simulink model "PoleCart"  (R2025a)
settings: Solver=ode23s  StartTime=0.0  StopTime=Tf  RelTol=1e-3  AbsTol=1e-3  EnableMultiTasking=on
model workspace (MAT data in the model file):
  Max_Trq = 10
values from neighbouring files (symbols this model uses):
  AncleDegLowerLim = -45    [PoleCart_ini.m]    (also in initialize_Parameters.m = Simulink.Parameter)
  AncleDegUpperLim = 45    [PoleCart_ini.m]    (also in initialize_Parameters.m = Simulink.Parameter)
  BallUnderFootRad = 1e-2    (= 0.01)    [PoleCart_ini.m]    (also in initialize_Parameters.m = Simulink.Parameter)
  FootX = 0.1    [PoleCart_ini.m]    (also in initialize_Parameters.m = Simulink.Parameter)
  FootY = 0.25    [PoleCart_ini.m]    (also in initialize_Parameters.m = Simulink.Parameter)
  FootZ = 0.06    [PoleCart_ini.m]    (also in initialize_Parameters.m = Simulink.Parameter)
  InitialCondition = []    [initialize_Parameters.m]
  TibiaZ = 0.4    [PoleCart_ini.m]    (also in initialize_Parameters.m = Simulink.Parameter)
undefined symbols (not defined in the file or in its folder): X, Y, Z
libraries: sm_lib x24, nesl_utility x14, simulink x2, rllib x1
settings Model: Creator=naoki  LastModifiedBy=naoki
settings SolverCC: AutoScaleAbsTol=off  AlgebraicLoopSolver=TrustRegion  MaxZcPerStep=1.0
settings DataIOCC: LimitDataPoints=on  MaxDataPoints=10000
settings OptimizationCC: ReuseModelBlockBuffer=off  LifeSpan=inf
settings DebuggingCC: UnconnectedInputMsg=warning  UnconnectedOutputMsg=warning  UnconnectedLineMsg=warning  AllowSymbolicDim=off  SubsystemReferenceDiagnosticForUnitTest=warning  SFUnexpectedBacktrackingDiag=warning  SFNoUnconditionalDefaultTransitionDiag=warning  SFExecutionAtInitializationDiag=none  ArithmeticOperatorsInVariantConditions=warning
settings ModelReferenceCC: EnableRefExpFcnMdlSchedulingChecks=on
settings SFSimCC: SimUseLocalCustomCode=off  CustomCodeUndefinedFunction=UseInterfaceOnly
settings RTWCC: RTWUseLocalCustomCode=off  GPUComputeCapability=3.5  DLArmComputeVersion=19.05
settings CodeAppCC: StateflowObjectComments=on
settings GRTTargetCC: TargetLangStandard=C89/C90 (ANSI)
settings ConfigComp: CovMetricSettings=dw  CovSaveCumulativeToWorkspaceVar=on  CovSaveSingleToWorkspaceVar=on  CovExternalEMLEnable=off  CovSFcnEnable=off
settings SimscapeCC: SimscapeLogType=all  SimscapeLogSimulationStatistics=on  SimscapeLogDataHistory=10000.0

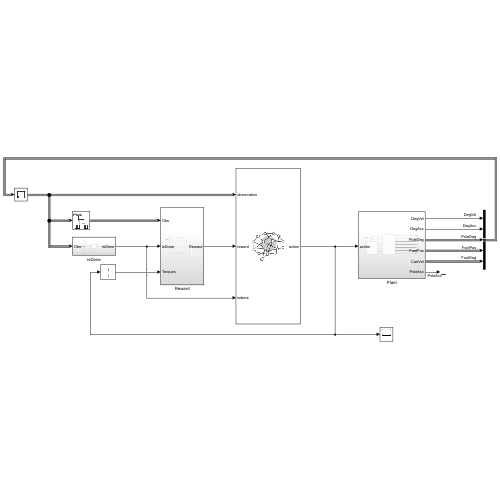
[thumbnail: Simulink's stored preview of the top-level diagram]
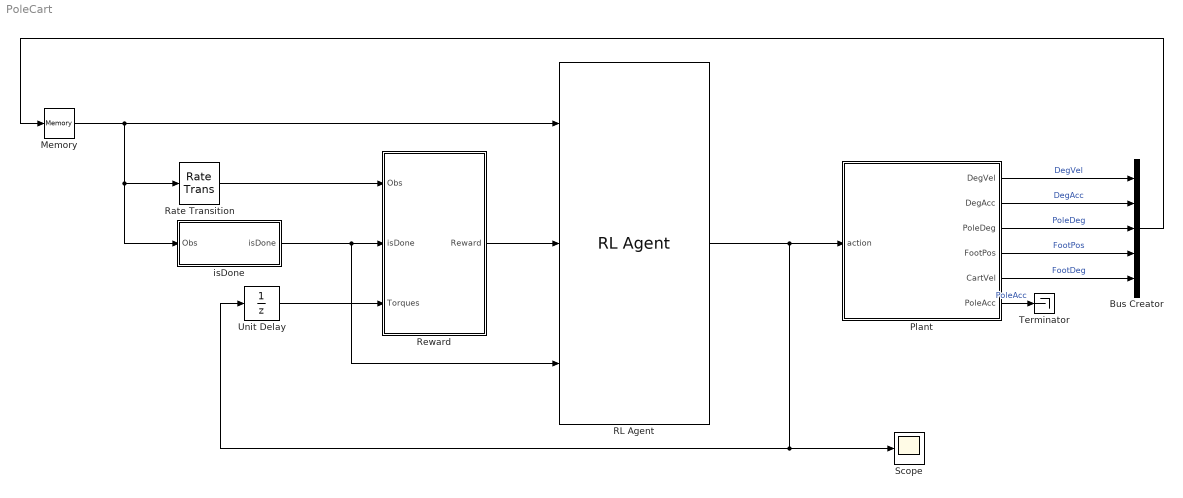
== system PoleCart ==
  Bus Creator : BusCreator  Inputs=5
  Memory : Memory  InitialCondition=InitialCondition
  Plant : Subsystem
  RL Agent : rllib/RL Agent  Agent=agentObj  ExternalActionAsInput=off  ProvideLastAction=off  ProvideCumRwd=off  TreatAsDirectFeedthrough=on  UseStrictObservationDataTypes=off
  Rate Transition : RateTransition  OutPortSampleTime=Ts
  Reward : Subsystem
  Scope : Scope
  Terminator : Terminator
  Unit Delay : UnitDelay  SampleTime=-1  HasFrameUpgradeWarning=on
  isDone : Subsystem
  wires:
  Plant/2(DegAcc) -> Bus Creator/2  "DegAcc"
  Plant/1(DegVel) -> Bus Creator/1  "DegVel"
  Memory/1 -> isDone/1(Obs), Rate Transition/1, RL Agent/1
  Reward/1(Reward) -> RL Agent/2
  isDone/1(isDone) -> RL Agent/3, Reward/2(isDone)
  Plant/3(PoleDeg) -> Bus Creator/3  "PoleDeg"
  Rate Transition/1 -> Reward/1(Obs)
  Plant/4(FootPos) -> Bus Creator/4  "FootPos"
  Plant/5(CartVel) -> Bus Creator/5  "FootDeg"
  Unit Delay/1 -> Reward/3(Torques)
  Bus Creator/1 -> Memory/1
  RL Agent/1 -> Scope/1, Unit Delay/1, Plant/1(action)
  Plant/6(PoleAcc) -> Terminator/1  "PoleAcc"

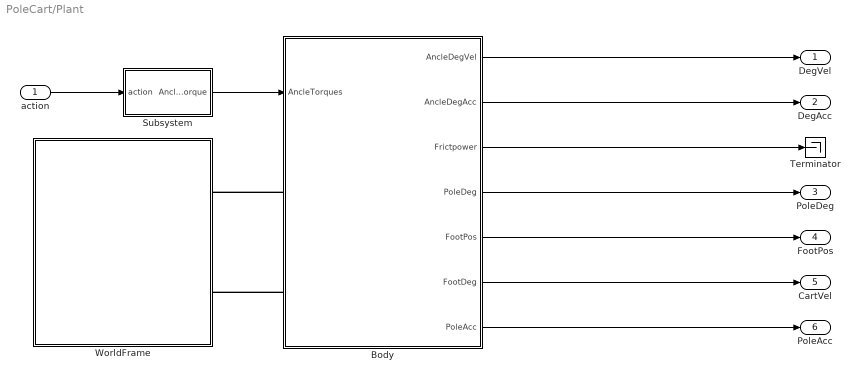
== system PoleCart/Plant ==
  action : Inport
  Body : Subsystem
  Subsystem : Subsystem
  Terminator : Terminator
  WorldFrame : Subsystem
  DegVel : Outport
  DegAcc : Outport  Port=2
  PoleDeg : Outport  Port=3
  FootPos : Outport  Port=4
  CartVel : Outport  Port=5
  PoleAcc : Outport  Port=6
  wires:
  Body/1(AncleDegVel) -> DegVel/1
  Body/2(AncleDegAcc) -> DegAcc/1
  Body/3(Frictpower) -> Terminator/1
  Body/4(PoleDeg) -> PoleDeg/1
  action/1 -> Subsystem/1(action)
  Subsystem/1(AncleTorque) -> Body/1(AncleTorques)
  Body/6(FootDeg) -> CartVel/1
  Body/5(FootPos) -> FootPos/1
  Body/7(PoleAcc) -> PoleAcc/1
  connections:
  Body/LConn1 -- WorldFrame/RConn1
  Body/LConn2 -- WorldFrame/RConn2

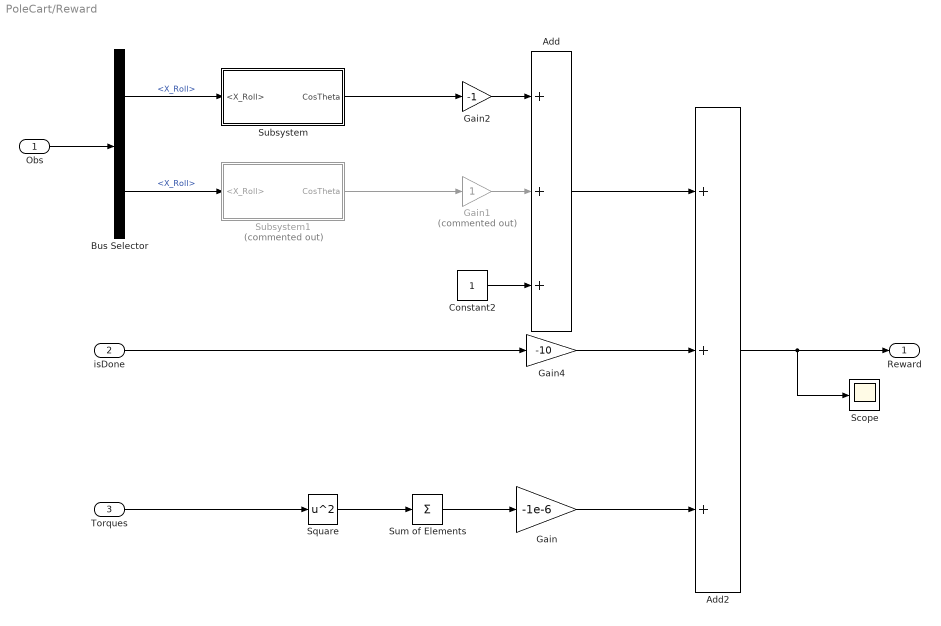
== system PoleCart/Reward ==
  Obs : Inport
  isDone : Inport  Port=2
  Torques : Inport  Port=3
  Add : Sum  Inputs=+++
  Add2 : Sum  Inputs=+++
  Bus Selector : BusSelector  OutputSignals=PoleDeg.X_Roll,FootDeg.X_Roll
  Constant2 : Constant
  Gain : Gain  Gain=-1e-6
  Gain1 : Gain  Commented=on
  Gain2 : Gain  Gain=-1
  Gain4 : Gain  Gain=-10
  Scope : Scope
      settings: ActiveDisplayYMinimum=0.87075945587495107  ActiveDisplayYMaximum=1.0142496566239427
  Square : Math  Operator=square
  Subsystem : Subsystem
  Subsystem1 : Subsystem  Commented=on
  Sum of Elements : Sum  Inputs=+
  Reward : Outport
  wires:
  Obs/1 -> Bus Selector/1
  Subsystem/1(CosTheta) -> Gain2/1
  Bus Selector/1 -> Subsystem/1(<X_Roll>)  "<X_Roll>"
  isDone/1 -> Gain4/1
  Constant2/1 -> Add/3
  Add/1 -> Add2/1
  Gain4/1 -> Add2/2
  Add2/1 -> Reward/1, Scope/1
  Torques/1 -> Square/1
  Square/1 -> Sum of Elements/1
  Sum of Elements/1 -> Gain/1
  Gain/1 -> Add2/3
  Gain2/1 -> Add/1
  Gain1/1 -> Add/2
  Bus Selector/2 -> Subsystem1/1(<X_Roll>)  "<X_Roll>"
  Subsystem1/1(CosTheta) -> Gain1/1

== system PoleCart/isDone ==
  Obs : Inport
  Bus Selector : BusSelector  OutputSignals=PoleDeg.X_Roll
  Subsystem : Subsystem
  isDone : Outport
  wires:
  Obs/1 -> Bus Selector/1
  Bus Selector/1 -> Subsystem/1(<X_Roll>)  "<X_Roll>"
  Subsystem/1(isDone) -> isDone/1

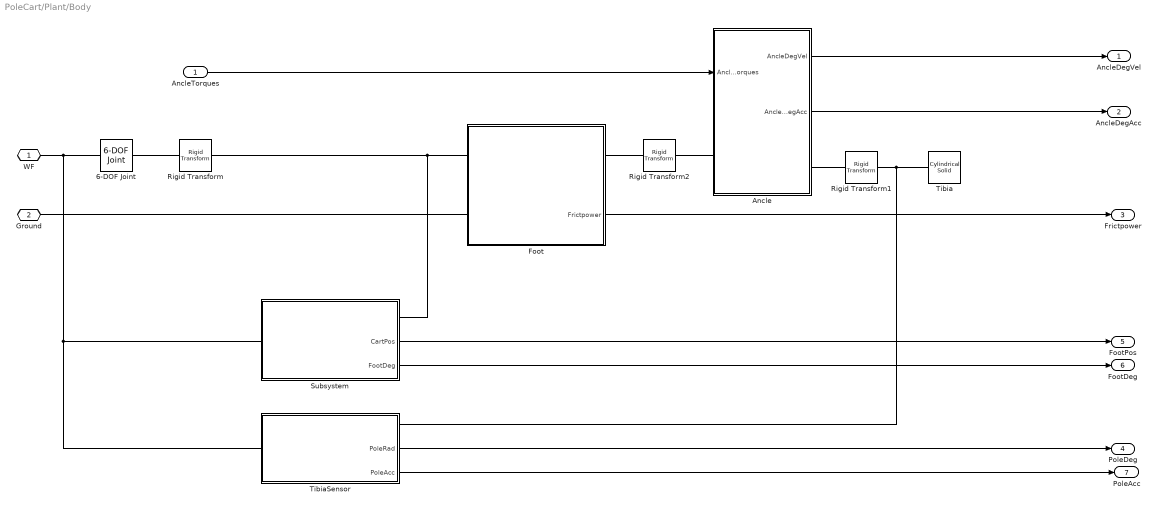
== system PoleCart/Plant/Body ==
  AncleTorques : Inport
  6-DOF Joint : sm_lib/Joints/6-DOF Joint  JointMode=Normal  CompositeWrenchDir=FollowerOnBase  CompositeWrenchFrame=BaseFrame  SenseConstraintForce=off  SenseConstraintTorque=off  SenseTotalForce=off  SenseTotalTorque=off  PxPositionTargetSpecify=off  PxPositionTargetPriority=High  PxPositionTargetValue=0  PxPositionTargetValueUnits=m  PxVelocityTargetSpecify=off  PxVelocityTargetPriority=High  PxVelocityTargetValue=0  PxVelocityTargetValueUnits=m/s  PxEquilibriumPosition=0  PxEquilibriumPositionUnits=m  PxSpringStiffness=0  PxSpringStiffnessUnits=N/m  PxDampingCoefficient=0  PxDampingCoefficientUnits=N/(m/s)  PxLowerLimitSpecify=off  PxLowerLimitBound=-1  PxLowerLimitBoundUnits=m  PxLowerLimitStiffness=1e6  PxLowerLimitStiffnessUnits=N/m  PxLowerLimitDamping=1e3  PxLowerLimitDampingUnits=N/(m/s)  PxLowerLimitTransitionRegionWidth=1e-4  PxLowerLimitTransitionRegionWidthUnits=m  PxUpperLimitSpecify=off  PxUpperLimitBound=1  PxUpperLimitBoundUnits=m  PxUpperLimitStiffness=1e6  PxUpperLimitStiffnessUnits=N/m  PxUpperLimitDamping=1e3  PxUpperLimitDampingUnits=N/(m/s)  PxUpperLimitTransitionRegionWidth=1e-4  PxUpperLimitTransitionRegionWidthUnits=m  PxTorqueActuationMode=NoTorque  PxMotionActuationMode=ComputedMotion  PxSensePosition=off  PxSenseVelocity=off  PxSenseAcceleration=off  PxSenseTorqueForce=off  PxSenseLowerLimitTorqueForce=off  PxSenseUpperLimitTorqueForce=off  PyPositionTargetSpecify=off  PyPositionTargetPriority=High  PyPositionTargetValue=0  PyPositionTargetValueUnits=m  PyVelocityTargetSpecify=off  PyVelocityTargetPriority=High  PyVelocityTargetValue=0  PyVelocityTargetValueUnits=m/s  PyEquilibriumPosition=0  PyEquilibriumPositionUnits=m  PySpringStiffness=0  PySpringStiffnessUnits=N/m  PyDampingCoefficient=0  PyDampingCoefficientUnits=N/(m/s)  PyLowerLimitSpecify=off  PyLowerLimitBound=-1  PyLowerLimitBoundUnits=m  PyLowerLimitStiffness=1e6  PyLowerLimitStiffnessUnits=N/m  PyLowerLimitDamping=1e3  PyLowerLimitDampingUnits=N/(m/s)  PyLowerLimitTransitionRegionWidth=1e-4  PyLowerLimitTransitionRegionWidthUnits=m  PyUpperLimitSpecify=off  PyUpperLimitBound=1  PyUpperLimitBoundUnits=m  PyUpperLimitStiffness=1e6  PyUpperLimitStiffnessUnits=N/m  PyUpperLimitDamping=1e3  PyUpperLimitDampingUnits=N/(m/s)  PyUpperLimitTransitionRegionWidth=1e-4  PyUpperLimitTransitionRegionWidthUnits=m  PyTorqueActuationMode=NoTorque  PyMotionActuationMode=ComputedMotion  PySensePosition=off  PySenseVelocity=off  PySenseAcceleration=off  PySenseTorqueForce=off  PySenseLowerLimitTorqueForce=off  PySenseUpperLimitTorqueForce=off  PzPositionTargetSpecify=off  PzPositionTargetPriority=High  PzPositionTargetValue=0  PzPositionTargetValueUnits=m  PzVelocityTargetSpecify=off  PzVelocityTargetPriority=High  PzVelocityTargetValue=0  PzVelocityTargetValueUnits=m/s  PzEquilibriumPosition=0  PzEquilibriumPositionUnits=m  PzSpringStiffness=0  PzSpringStiffnessUnits=N/m  PzDampingCoefficient=0  PzDampingCoefficientUnits=N/(m/s)  PzLowerLimitSpecify=off  PzLowerLimitBound=-1  PzLowerLimitBoundUnits=m  PzLowerLimitStiffness=1e6  PzLowerLimitStiffnessUnits=N/m  PzLowerLimitDamping=1e3  PzLowerLimitDampingUnits=N/(m/s)  PzLowerLimitTransitionRegionWidth=1e-4  PzLowerLimitTransitionRegionWidthUnits=m  PzUpperLimitSpecify=off  PzUpperLimitBound=1  PzUpperLimitBoundUnits=m  PzUpperLimitStiffness=1e6  PzUpperLimitStiffnessUnits=N/m  PzUpperLimitDamping=1e3  PzUpperLimitDampingUnits=N/(m/s)  PzUpperLimitTransitionRegionWidth=1e-4  PzUpperLimitTransitionRegionWidthUnits=m  PzTorqueActuationMode=NoTorque  PzMotionActuationMode=ComputedMotion  PzSensePosition=off  PzSenseVelocity=off  PzSenseAcceleration=off  PzSenseTorqueForce=off  PzSenseLowerLimitTorqueForce=off  PzSenseUpperLimitTorqueForce=off  SphPositionTargetSpecify=off  SphPositionTargetPriority=High  SphPositionTargetRotationMethod=None  SphPositionTargetFollAlignAxisA=+X  SphPositionTargetBaseAlignAxisA=+Y  SphPositionTargetFollAlignAxisB=+Y  SphPositionTargetBaseAlignAxisB=+Z  SphPositionTargetRotationStandardAxis=+Z  SphPositionTargetRotationAngle=0  SphPositionTargetRotationAngleUnits=deg  SphPositionTargetRotationArbitraryAxis=[0 0 1]  SphPositionTargetRotationSequenceAxes=FollowerAxes  SphPositionTargetRotationSequence=XYX  SphPositionTargetRotationSequenceAngles=[0 0 0]  SphPositionTargetRotationSequenceAnglesUnits=deg  SphPositionTargetRotationMatrix=[1 0 0;0 1 0;0 0 1]  SphPositionTargetQuaternion=[1 0 0 0]  SphVelocityTargetSpecify=off  SphVelocityTargetPriority=High  SphVelocityTargetValue=[0 0 0]  SphVelocityTargetValueUnits=deg/s  SphVelocityTargetInFollowerFrame=on  SphEqPosRotationMethod=None  SphEqPosFollAlignAxisA=+X  SphEqPosBaseAlignAxisA=+Y  SphEqPosFollAlignAxisB=+Y  SphEqPosBaseAlignAxisB=+Z  SphEqPosRotationStandardAxis=+Z  SphEqPosRotationAngle=0  SphEqPosRotationAngleUnits=deg  SphEqPosRotationArbitraryAxis=[0 0 1]  SphEqPosRotationSequenceAxes=FollowerAxes  SphEqPosRotationSequence=XYX  SphEqPosRotationSequenceAngles=[0 0 0]  SphEqPosRotationSequenceAnglesUnits=deg  SphEqPosRotationMatrix=[1 0 0;0 1 0;0 0 1]  SphEqPosQuaternion=[1 0 0 0]  SphSpringStiffness=0  SphSpringStiffnessUnits=N*m/deg  SphDampingCoefficient=0  SphDampingCoefficientUnits=N*m/(deg/s)  SphLowerLimitSpecify=off  SphLowerLimitBound=15  SphLowerLimitBoundUnits=deg  SphLowerLimitStiffness=1e4  SphLowerLimitStiffnessUnits=N*m/deg  SphLowerLimitDamping=10  SphLowerLimitDampingUnits=N*m/(deg/s)  SphLowerLimitTransitionRegionWidth=0.1  SphLowerLimitTransitionRegionWidthUnits=deg  SphUpperLimitSpecify=off  SphUpperLimitBound=45  SphUpperLimitBoundUnits=deg  SphUpperLimitStiffness=1e4  SphUpperLimitStiffnessUnits=N*m/deg  SphUpperLimitDamping=10  SphUpperLimitDampingUnits=N*m/(deg/s)  SphUpperLimitTransitionRegionWidth=0.1  SphUpperLimitTransitionRegionWidthUnits=deg  SphTorqueActuationMode=NoTorque  SphActuateTorqueX=off  SphActuateTorqueY=off  SphActuateTorqueZ=off  SphActuateTorque=off  SphActuationFrame=BaseFrame  SphSensePosition=off  SphSenseVelocityX=off  SphSenseVelocityY=off  SphSenseVelocityZ=off  SphSenseVelocity=off  SphSenseAccelerationX=off  SphSenseAccelerationY=off  SphSenseAccelerationZ=off  SphSenseAcceleration=off  SphSenseLowerLimitTorqueMag=off  SphSenseUpperLimitTorqueMag=off  SphSensingFrame=BaseFrame
  Ancle : Subsystem
  Foot : Subsystem
      settings: PortSchema="{\"entries\":[{\"content\":{\"sides\":[{\"content\":{\"connectorIds\":[\"LConn1\",\"LConn2\"]},\"type\":\"ConnectorPlacement.EquallySpacedRectSide\",\"uuid\":\"d5f97005-16a4-49fe-94e6-d10e7af0ba01\"},{\"content\":{\"connectorIds\":[\"RConn1\",\"Out1\"],\"side\":\"RIGHT\"},\"type\":\"ConnectorPlacement.EquallySpacedRectSide\",\"uuid\":\"9f5dca56-320d-4a75-a909-fa3bd9aed5d9\"},{\"content\":{\"side\":\"TOP\"},\"type\":\"ConnectorPlacement.EquallySpacedRectSide\",\"uuid\":\"63cf01ef-a1c2-47e2-84ff-3fab955ff73c\"}]},\"type\":\"ConnectorPlacement.EquallySpacedConnector\",\"uuid\":\"bd2d193d-b664-4209-9b54-5802503f6a3c\"}],\"packageUris\":[\"http://schema.mathworks.com/mf0/Connector/R2020b\"],\"version\":\"1.0\"}"
  Rigid Transform : sm_lib/Frames and Transforms/Rigid Transform  RotationMethod=None  FollAlignAxisA=+X  BaseAlignAxisA=+Y  FollAlignAxisB=+Y  BaseAlignAxisB=+Z  RotationStandardAxis=+Z  RotationAngle=0.0  RotationAngleUnits=deg  RotationArbitraryAxis=[0 0 1]  RotationSequenceAxes=FollowerAxes  RotationSequence=XYX  RotationSequenceAngles=[0 0 0]  RotationSequenceAnglesUnits=deg  RotationMatrix=[1 0 0; 0 1 0; 0 0 1]  Quaternion=[1 0 0 0]  TranslationMethod=StandardAxis  TranslationCartesianOffset=[0 0 0]  TranslationCartesianOffsetUnits=m  TranslationStandardAxis=+Z  TranslationStandardOffset=FootZ/2 + 2*BallUnderFootRad  TranslationStandardOffsetUnits=m  TranslationROffset=0  TranslationROffsetUnits=m  TranslationThetaOffset=0  TranslationThetaOffsetUnits=deg  TranslationZOffset=0  TranslationZOffsetUnits=m
  Rigid Transform1 : sm_lib/Frames and Transforms/Rigid Transform  RotationMethod=StandardAxis  FollAlignAxisA=+X  BaseAlignAxisA=+Y  FollAlignAxisB=+Y  BaseAlignAxisB=+Z  RotationStandardAxis=+Y  RotationAngle=90  RotationAngleUnits=deg  RotationArbitraryAxis=[0 0 1]  RotationSequenceAxes=FollowerAxes  RotationSequence=XYX  RotationSequenceAngles=[0 0 0]  RotationSequenceAnglesUnits=deg  RotationMatrix=[1 0 0; 0 1 0; 0 0 1]  Quaternion=[1 0 0 0]  TranslationMethod=StandardAxis  TranslationCartesianOffset=[0 0 0]  TranslationCartesianOffsetUnits=m  TranslationStandardAxis=+X  TranslationStandardOffset=TibiaZ/2  TranslationStandardOffsetUnits=m  TranslationROffset=0  TranslationROffsetUnits=m  TranslationThetaOffset=0  TranslationThetaOffsetUnits=deg  TranslationZOffset=0  TranslationZOffsetUnits=m
  Rigid Transform2 : sm_lib/Frames and Transforms/Rigid Transform  RotationMethod=StandardAxis  FollAlignAxisA=+X  BaseAlignAxisA=+Y  FollAlignAxisB=+Y  BaseAlignAxisB=+Z  RotationStandardAxis=+Y  RotationAngle=-90  RotationAngleUnits=deg  RotationArbitraryAxis=[0 0 1]  RotationSequenceAxes=FollowerAxes  RotationSequence=XYX  RotationSequenceAngles=[0 0 0]  RotationSequenceAnglesUnits=deg  RotationMatrix=[1 0 0; 0 1 0; 0 0 1]  Quaternion=[1 0 0 0]  TranslationMethod=StandardAxis  TranslationCartesianOffset=[0 0 0]  TranslationCartesianOffsetUnits=m  TranslationStandardAxis=+Z  TranslationStandardOffset=FootZ/2  TranslationStandardOffsetUnits=m  TranslationROffset=0  TranslationROffsetUnits=m  TranslationThetaOffset=0  TranslationThetaOffsetUnits=deg  TranslationZOffset=0  TranslationZOffsetUnits=m
  Subsystem : Subsystem
      settings: PortSchema="{\"entries\":[{\"content\":{\"sides\":[{\"content\":{\"connectorIds\":[\"LConn1\",\"Out1\",\"Out2\"]},\"type\":\"ConnectorPlacement.EquallySpacedRectSide\",\"uuid\":\"005876bf-2c81-461b-a6bd-4eb35ecb173d\"},{\"content\":{\"connectorIds\":[\"RConn1\"],\"side\":\"RIGHT\"},\"type\":\"ConnectorPlacement.EquallySpacedRectSide\",\"uuid\":\"4a0b3e71-b49d-4262-b788-0100c2880398\"},{\"content\":{\"side\":\"TOP\"},\"type\":\"ConnectorPlacement.EquallySpacedRectSide\",\"uuid\":\"bd0622e9-063e-46ae-b2fe-36cbf237fb6a\"}]},\"type\":\"ConnectorPlacement.EquallySpacedConnector\",\"uuid\":\"4a00f615-6add-406e-8a2c-6a8c2c2b8412\"}],\"packageUris\":[\"http://schema.mathworks.com/mf0/Connector/R2020b\"],\"version\":\"1.0\"}"
  Tibia : sm_lib/Body Elements/Cylindrical Solid  CylinderRadius=TibiaX  CylinderRadiusUnits=m  CylinderLength=TibiaZ  CylinderLengthUnits=m  ExportEntireGeometry=off  InertiaType=CalculateFromGeometry  BasedOnType=Density  Density=TibiaDencity  DensityUnits=kg/m^3  Mass=1  MassUnits=kg  CenterOfMass=[0 0 0]  CenterOfMassUnits=m  MomentsOfInertia=[1 1 1]  MomentsOfInertiaUnits=kg*m^2  ProductsOfInertia=[0 0 0]  ProductsOfInertiaUnits=kg*m^2  GraphicType=FromGeometry  MarkerShape=Sphere  MarkerSize=10  GraphicVisPropType=SimpleVisualProperties  GraphicDiffuseColor=[0.5 0.5 0.5]  GraphicOpacity=1  GraphicSpecularColor=[0.5 0.5 0.5 1.0]  GraphicAmbientColor=[0.15 0.15 0.15 1.0]  GraphicEmissiveColor=[0.0 0.0 0.0 1.0]  GraphicShininess=75  DoExposeReferenceFrame=on  SerializedFrames=<Frames/>
  TibiaSensor : Subsystem
      settings: PortSchema="{\"entries\":[{\"content\":{\"sides\":[{\"content\":{\"connectorIds\":[\"LConn1\"]},\"type\":\"ConnectorPlacement.EquallySpacedRectSide\",\"uuid\":\"f3ebb2df-a6b1-403e-80ba-08f1b279a761\"},{\"content\":{\"connectorIds\":[\"RConn1\",\"Out1\",\"Out2\"],\"side\":\"RIGHT\"},\"type\":\"ConnectorPlacement.EquallySpacedRectSide\",\"uuid\":\"e83d7573-3688-496f-bb9e-845594156150\"},{\"content\":{\"side\":\"TOP\"},\"type\":\"ConnectorPlacement.EquallySpacedRectSide\",\"uuid\":\"3eeef0ea-f381-4ec1-9671-20ff7e8b50b6\"}]},\"type\":\"ConnectorPlacement.EquallySpacedConnector\",\"uuid\":\"b1f4614b-fa2d-4bb0-ae56-925dd51b275d\"}],\"packageUris\":[\"http://schema.mathworks.com/mf0/Connector/R2020b\"],\"version\":\"1.0\"}"
  WF : PMIOPort  Side=Left
  Ground : PMIOPort  Port=2  Side=Left
  AncleDegVel : Outport
  AncleDegAcc : Outport  Port=2
  Frictpower : Outport  Port=3
  PoleDeg : Outport  Port=4
  FootPos : Outport  Port=5
  FootDeg : Outport  Port=6
  PoleAcc : Outport  Port=7
  wires:
  AncleTorques/1 -> Ancle/1(AncleTorques)
  Ancle/2(AncleDegAcc) -> AncleDegAcc/1
  Foot/1(Frictpower) -> Frictpower/1
  Ancle/1(AncleDegVel) -> AncleDegVel/1
  TibiaSensor/1(PoleRad) -> PoleDeg/1
  Subsystem/1(CartPos) -> FootPos/1
  Subsystem/2(FootDeg) -> FootDeg/1
  TibiaSensor/2(PoleAcc) -> PoleAcc/1
  connections:
  Ancle/LConn1 -- Rigid Transform2/RConn1
  Rigid Transform/LConn1 -- 6-DOF Joint/RConn1
  Tibia/RConn1 -- TibiaSensor/RConn1 -- Rigid Transform1/RConn1
  Foot/LConn1 -- Subsystem/LConn1 -- Rigid Transform/RConn1
  Rigid Transform2/LConn1 -- Foot/RConn1
  Rigid Transform1/LConn1 -- Ancle/RConn1
  Foot/LConn2 -- Ground/RConn1
  6-DOF Joint/LConn1 -- Subsystem/RConn1 -- TibiaSensor/LConn1 -- WF/RConn1

== system PoleCart/Plant/Subsystem ==
  action : Inport
  Selector : Selector  InputPortWidth=1  IndexOptions=Index vector (dialog)  Indices=1  OutputSizes=1
  AncleTorque : Outport
  wires:
  Selector/1 -> AncleTorque/1
  action/1 -> Selector/1

== system PoleCart/Plant/WorldFrame ==
  Infinite Plane : sm_lib/Curves and Surfaces/Infinite Plane  GraphicType=Rectangle  GraphicPlaneWidth=1  GraphicPlaneWidthUnits=m  GraphicPlaneHeight=1  GraphicPlaneHeightUnits=m  GraphicVisPropType=SimpleVisualProperties  GraphicDiffuseColor=[0.5 0.5 0.5]  GraphicOpacity=1  GraphicSpecularColor=[0.5 0.5 0.5 1.0]  GraphicAmbientColor=[0.15 0.15 0.15 1.0]  GraphicEmissiveColor=[0.0 0.0 0.0 1.0]  GraphicShininess=75
  Subsystem2 : Subsystem
  WF : PMIOPort  Side=Right
  Ground : PMIOPort  Port=2  Side=Right
  connections:
  Infinite Plane/LConn1 -- WF/RConn1 -- Subsystem2/RConn1
  Ground/RConn1 -- Infinite Plane/RConn1

== system PoleCart/Reward/Subsystem ==
  <X_Roll> : Inport
  Abs : Abs  SaturateOnIntegerOverflow=off
  Cos : Trigonometry
  Gain : Gain  Gain=180/pi
  Scope : Scope  NumInputPorts=2
      settings: ActiveDisplayYMinimum=-50.307423277470271  ActiveDisplayYMaximum=0.20034172662394845  DataLoggingVariableName=ScopeData6
  CosTheta : Outport
  wires:
  Cos/1 -> Abs/1
  <X_Roll>/1 -> Gain/1, Cos/1
  Gain/1 -> Scope/1
  Abs/1 -> Scope/2, CosTheta/1

== system PoleCart/Reward/Subsystem1 ==
  <X_Roll> : Inport
  Cos : Trigonometry  Operator=cos
  CosTheta : Outport
  wires:
  Cos/1 -> CosTheta/1
  <X_Roll>/1 -> Cos/1

== system PoleCart/isDone/Subsystem ==
  <X_Roll> : Inport
  Compare To Constant : simulink/Logic and Bit Operations/Compare To Constant  relop=>=  const=AncleDegUpperLim  OutDataTypeStr=boolean
  Compare To Constant1 : simulink/Logic and Bit Operations/Compare To Constant  relop=<=  const=AncleDegLowerLim  OutDataTypeStr=boolean
  Gain : Gain  Gain=180/pi
  Logical Operator : Logic  Operator=OR  AllPortsSameDT=off  OutDataTypeStr=boolean
  isDone : Outport
  wires:
  <X_Roll>/1 -> Gain/1
  Compare To Constant1/1 -> Logical Operator/2
  Compare To Constant/1 -> Logical Operator/1
  Logical Operator/1 -> isDone/1
  Gain/1 -> Compare To Constant1/1, Compare To Constant/1

== system PoleCart/Plant/Body/Ancle ==
  AncleTorques : Inport
  PS-Simulink Converter1 : nesl_utility/PS-Simulink Converter  PhysicalDomain=network_engine_domain  SubClassName=ps_output  LeftPortType=input  RightPortType=output  PseudoPeriodic=off  Frequencies=[]  VectorFormat=inherit  Unit=inherit  AffineConversion=off
  PS-Simulink Converter2 : nesl_utility/PS-Simulink Converter  PhysicalDomain=network_engine_domain  SubClassName=ps_output  LeftPortType=input  RightPortType=output  PseudoPeriodic=off  Frequencies=[]  VectorFormat=inherit  Unit=inherit  AffineConversion=off
  Revolute Joint : sm_lib/Joints/Revolute Joint  JointMode=Normal  CompositeWrenchDir=FollowerOnBase  CompositeWrenchFrame=BaseFrame  SenseConstraintForce=off  SenseConstraintTorque=off  SenseTotalForce=off  SenseTotalTorque=off  PositionTargetSpecify=on  PositionTargetPriority=High  PositionTargetValue=AncleDegInit  PositionTargetValueUnits=deg  VelocityTargetSpecify=off  VelocityTargetPriority=High  VelocityTargetValue=AncleTorqueInit  VelocityTargetValueUnits=deg/s  EquilibriumPosition=0  EquilibriumPositionUnits=deg  SpringStiffness=0  SpringStiffnessUnits=N*m/deg  DampingCoefficient=0  DampingCoefficientUnits=N*m/(deg/s)  LowerLimitSpecify=on  LowerLimitBound=AncleDegLowerLim  LowerLimitBoundUnits=deg  LowerLimitStiffness=1e4  LowerLimitStiffnessUnits=N*m/deg  LowerLimitDamping=10  LowerLimitDampingUnits=N*m/(deg/s)  LowerLimitTransitionRegionWidth=0.1  LowerLimitTransitionRegionWidthUnits=deg  UpperLimitSpecify=on  UpperLimitBound=AncleDegUpperLim  UpperLimitBoundUnits=deg  UpperLimitStiffness=1e4  UpperLimitStiffnessUnits=N*m/deg  UpperLimitDamping=10  UpperLimitDampingUnits=N*m/(deg/s)  UpperLimitTransitionRegionWidth=0.1  UpperLimitTransitionRegionWidthUnits=deg  TorqueActuationMode=InputTorque  MotionActuationMode=ComputedMotion  SensePosition=off  SenseVelocity=on  SenseAcceleration=on  SenseTorqueForce=off  SenseLowerLimitTorqueForce=off  SenseUpperLimitTorqueForce=off
  Simulink-PS Converter : nesl_utility/Simulink-PS Converter  PhysicalDomain=network_engine_domain  SubClassName=ps_input  LeftPortType=input  RightPortType=output  PseudoPeriodic=off  Frequencies=[]  NoiseDistribution=none  NoiseParameters=[]  Unit=1  AffineConversion=off  FilteringAndDerivatives=provide  SimscapeFilterOrder=1  InputFilterTimeConstant=0.001  UdotUserProvided=0
  Ancle : PMIOPort  Side=Right
  Foot : PMIOPort  Port=2  Side=Left
  AncleDegVel : Outport
  AncleDegAcc : Outport  Port=2
  wires:
  AncleTorques/1 -> Simulink-PS Converter/1
  PS-Simulink Converter1/1 -> AncleDegVel/1
  PS-Simulink Converter2/1 -> AncleDegAcc/1
  connections:
  Ancle/RConn1 -- Revolute Joint/RConn1
  Simulink-PS Converter/RConn1 -- Revolute Joint/LConn2
  PS-Simulink Converter2/LConn1 -- Revolute Joint/RConn3
  PS-Simulink Converter1/LConn1 -- Revolute Joint/RConn2
  Revolute Joint/LConn1 -- Foot/RConn1

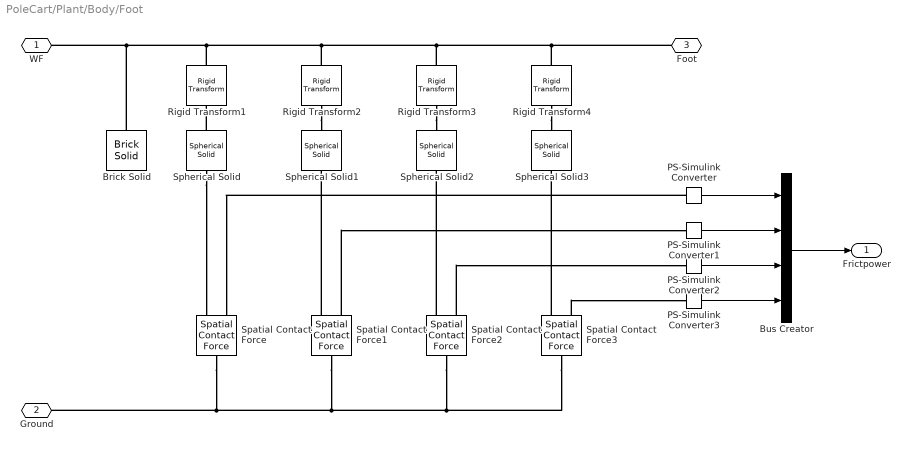
== system PoleCart/Plant/Body/Foot ==
  Brick Solid : sm_lib/Body Elements/Brick Solid  BrickDimensions=[FootX FootY FootZ]  BrickDimensionsUnits=m  ExportEntireGeometry=off  InertiaType=CalculateFromGeometry  BasedOnType=Density  Density=FootDencity  DensityUnits=kg/m^3  Mass=1  MassUnits=kg  CenterOfMass=[0 0 0]  CenterOfMassUnits=m  MomentsOfInertia=[1 1 1]  MomentsOfInertiaUnits=kg*m^2  ProductsOfInertia=[0 0 0]  ProductsOfInertiaUnits=kg*m^2  GraphicType=FromGeometry  MarkerShape=Sphere  MarkerSize=10  GraphicVisPropType=SimpleVisualProperties  GraphicDiffuseColor=[0.5 0.5 0.5]  GraphicOpacity=1.0  GraphicSpecularColor=[0.5 0.5 0.5 1.0]  GraphicAmbientColor=[0.15 0.15 0.15 1.0]  GraphicEmissiveColor=[0.0 0.0 0.0 1.0]  GraphicShininess=75  DoExposeReferenceFrame=on  SerializedFrames=<Frames/>
  Bus Creator : BusCreator  Inputs=4
  PS-Simulink Converter{,1..3} (4 alike) : nesl_utility/PS-Simulink Converter  PhysicalDomain=network_engine_domain  SubClassName=ps_output  LeftPortType=input  RightPortType=output  PseudoPeriodic=off  Frequencies=[]  VectorFormat=inherit  Unit=inherit  AffineConversion=off
  Rigid Transform1 : sm_lib/Frames and Transforms/Rigid Transform  RotationMethod=None  FollAlignAxisA=+X  BaseAlignAxisA=+Y  FollAlignAxisB=+Y  BaseAlignAxisB=+Z  RotationStandardAxis=+Z  RotationAngle=0.0  RotationAngleUnits=deg  RotationArbitraryAxis=[0 0 1]  RotationSequenceAxes=FollowerAxes  RotationSequence=XYX  RotationSequenceAngles=[0 0 0]  RotationSequenceAnglesUnits=deg  RotationMatrix=[1 0 0; 0 1 0; 0 0 1]  Quaternion=[1 0 0 0]  TranslationMethod=Cartesian  TranslationCartesianOffset=[FootX/2 FootY/2 -FootZ/2]  TranslationCartesianOffsetUnits=m  TranslationStandardAxis=+Z  TranslationStandardOffset=FootZ/2  TranslationStandardOffsetUnits=m  TranslationROffset=0  TranslationROffsetUnits=m  TranslationThetaOffset=0  TranslationThetaOffsetUnits=deg  TranslationZOffset=0  TranslationZOffsetUnits=m
  Rigid Transform2 : sm_lib/Frames and Transforms/Rigid Transform  RotationMethod=None  FollAlignAxisA=+X  BaseAlignAxisA=+Y  FollAlignAxisB=+Y  BaseAlignAxisB=+Z  RotationStandardAxis=+Z  RotationAngle=0.0  RotationAngleUnits=deg  RotationArbitraryAxis=[0 0 1]  RotationSequenceAxes=FollowerAxes  RotationSequence=XYX  RotationSequenceAngles=[0 0 0]  RotationSequenceAnglesUnits=deg  RotationMatrix=[1 0 0; 0 1 0; 0 0 1]  Quaternion=[1 0 0 0]  TranslationMethod=Cartesian  TranslationCartesianOffset=[FootX/2 -FootY/2 -FootZ/2]  TranslationCartesianOffsetUnits=m  TranslationStandardAxis=+Z  TranslationStandardOffset=FootZ/2  TranslationStandardOffsetUnits=m  TranslationROffset=0  TranslationROffsetUnits=m  TranslationThetaOffset=0  TranslationThetaOffsetUnits=deg  TranslationZOffset=0  TranslationZOffsetUnits=m
  Rigid Transform3 : sm_lib/Frames and Transforms/Rigid Transform  RotationMethod=None  FollAlignAxisA=+X  BaseAlignAxisA=+Y  FollAlignAxisB=+Y  BaseAlignAxisB=+Z  RotationStandardAxis=+Z  RotationAngle=0.0  RotationAngleUnits=deg  RotationArbitraryAxis=[0 0 1]  RotationSequenceAxes=FollowerAxes  RotationSequence=XYX  RotationSequenceAngles=[0 0 0]  RotationSequenceAnglesUnits=deg  RotationMatrix=[1 0 0; 0 1 0; 0 0 1]  Quaternion=[1 0 0 0]  TranslationMethod=Cartesian  TranslationCartesianOffset=[-FootX/2 FootY/2 -FootZ/2]  TranslationCartesianOffsetUnits=m  TranslationStandardAxis=+Z  TranslationStandardOffset=FootZ/2  TranslationStandardOffsetUnits=m  TranslationROffset=0  TranslationROffsetUnits=m  TranslationThetaOffset=0  TranslationThetaOffsetUnits=deg  TranslationZOffset=0  TranslationZOffsetUnits=m
  Rigid Transform4 : sm_lib/Frames and Transforms/Rigid Transform  RotationMethod=None  FollAlignAxisA=+X  BaseAlignAxisA=+Y  FollAlignAxisB=+Y  BaseAlignAxisB=+Z  RotationStandardAxis=+Z  RotationAngle=0.0  RotationAngleUnits=deg  RotationArbitraryAxis=[0 0 1]  RotationSequenceAxes=FollowerAxes  RotationSequence=XYX  RotationSequenceAngles=[0 0 0]  RotationSequenceAnglesUnits=deg  RotationMatrix=[1 0 0; 0 1 0; 0 0 1]  Quaternion=[1 0 0 0]  TranslationMethod=Cartesian  TranslationCartesianOffset=[-FootX/2 -FootY/2 -FootZ/2]  TranslationCartesianOffsetUnits=m  TranslationStandardAxis=+Z  TranslationStandardOffset=FootZ/2  TranslationStandardOffsetUnits=m  TranslationROffset=0  TranslationROffsetUnits=m  TranslationThetaOffset=0  TranslationThetaOffsetUnits=deg  TranslationZOffset=0  TranslationZOffsetUnits=m
  Spatial Contact Force{,1..3} (4 alike) : sm_lib/Forces and Torques/Spatial Contact Force  SenseSeparationDistance=off  NormalForceType=SmoothSpringDamper  NormalStiffness=Stiffness  NormalStiffnessUnits=N/m  NormalDamping=Damping  NormalDampingUnits=N/(m/s)  NormalTransitionRegionWidth=TRW  NormalTransitionRegionWidthUnits=m  FrictionType=SmoothStickSlip  CoefficientOfStaticFriction=0.5  CoefficientOfDynamicFriction=0.3  FrictionalCriticalVelocity=1e-3  FrictionalCriticalVelocityUnits=m/s  SenseContactSignal=off  SensePenetrationDepth=off  SenseNormalVelocity=off  SenseTangentialVelocity=off  SensingForceTorqueDirection=BaseOnFollower  SensingForceTorqueResolutionFrame=ContactFrame  SenseNormalForce=on  SenseNormalForceMagnitude=off  SenseNormalTorque=off  SenseFrictionalForce=off  SenseFrictionalForceMagnitude=off  SenseFrictionalTorque=off  SenseTotalForce=off  SenseTotalTorque=off  SenseContactBaseRotation=off  SenseContactBaseTranslation=off  SenseContactFollowerRotation=off  SenseContactFollowerTranslation=off  ZeroCrossDetectContactStartAndEnd=off
  Spherical Solid{,1..3} (4 alike) : sm_lib/Body Elements/Spherical Solid  SphereRadius=BallUnderFootRad  SphereRadiusUnits=m  ExportEntireGeometry=on  InertiaType=CalculateFromGeometry  BasedOnType=Density  Density=1000  DensityUnits=kg/m^3  Mass=1  MassUnits=kg  CenterOfMass=[0 0 0]  CenterOfMassUnits=m  MomentsOfInertia=[1 1 1]  MomentsOfInertiaUnits=kg*m^2  ProductsOfInertia=[0 0 0]  ProductsOfInertiaUnits=kg*m^2  GraphicType=FromGeometry  MarkerShape=Sphere  MarkerSize=10  GraphicVisPropType=SimpleVisualProperties  GraphicDiffuseColor=[0.5 0.5 0.5]  GraphicOpacity=1  GraphicSpecularColor=[0.5 0.5 0.5 1.0]  GraphicAmbientColor=[0.15 0.15 0.15 1.0]  GraphicEmissiveColor=[0.0 0.0 0.0 1.0]  GraphicShininess=75  DoExposeReferenceFrame=on  SerializedFrames=<Frames/>
  WF : PMIOPort  Side=Left
  Ground : PMIOPort  Port=2  Side=Left
  Foot : PMIOPort  Port=3  Side=Right
  Frictpower : Outport
  wires:
  PS-Simulink Converter3/1 -> Bus Creator/4
  PS-Simulink Converter2/1 -> Bus Creator/3
  PS-Simulink Converter1/1 -> Bus Creator/2
  PS-Simulink Converter/1 -> Bus Creator/1
  Bus Creator/1 -> Frictpower/1
  connections:
  Rigid Transform2/RConn1 -- Spherical Solid1/RConn1
  Brick Solid/RConn1 -- Rigid Transform2/LConn1 -- Rigid Transform3/LConn1 -- Rigid Transform4/LConn1 -- Foot/RConn1 -- Rigid Transform1/LConn1 -- WF/RConn1
  Spatial Contact Force2/RConn1 -- Spherical Solid2/LConn1
  Spatial Contact Force3/RConn1 -- Spherical Solid3/LConn1
  Spatial Contact Force/LConn1 -- Ground/RConn1 -- Spatial Contact Force1/LConn1 -- Spatial Contact Force3/LConn1 -- Spatial Contact Force2/LConn1
  Rigid Transform3/RConn1 -- Spherical Solid2/RConn1
  Spherical Solid/LConn1 -- Spatial Contact Force/RConn1
  Spatial Contact Force1/RConn1 -- Spherical Solid1/LConn1
  Spherical Solid/RConn1 -- Rigid Transform1/RConn1
  Rigid Transform4/RConn1 -- Spherical Solid3/RConn1
  PS-Simulink Converter/LConn1 -- Spatial Contact Force/RConn2
  Spatial Contact Force1/RConn2 -- PS-Simulink Converter1/LConn1
  Spatial Contact Force2/RConn2 -- PS-Simulink Converter2/LConn1
  Spatial Contact Force3/RConn2 -- PS-Simulink Converter3/LConn1

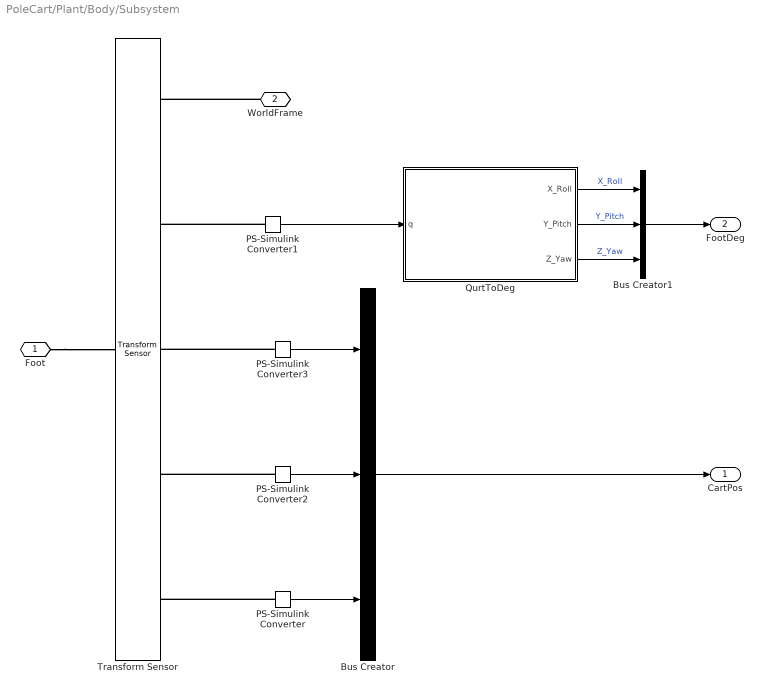
== system PoleCart/Plant/Body/Subsystem ==
  Bus Creator : BusCreator  Inputs=3
  Bus Creator1 : BusCreator  Inputs=3
  PS-Simulink Converter{,1..3} (4 alike) : nesl_utility/PS-Simulink Converter  PhysicalDomain=network_engine_domain  SubClassName=ps_output  LeftPortType=input  RightPortType=output  PseudoPeriodic=off  Frequencies=[]  VectorFormat=inherit  Unit=inherit  AffineConversion=off
  QurtToDeg : Subsystem
  Transform Sensor : sm_lib/Frames and Transforms/Transform Sensor  MeasurementFrame=World  RotationSequence=ZYX  SenseAngle=off  SenseAxis=off  SenseQ=on  SenseR=off  SenseRotationSequence=off  SenseOmegaX=off  SenseOmegaY=off  SenseOmegaZ=off  SenseOmega=off  SenseQDot=off  SenseRDot=off  SenseRotationSequenceDot=off  SenseAlphaX=off  SenseAlphaY=off  SenseAlphaZ=off  SenseAlpha=off  SenseQDDot=off  SenseRDDot=off  SenseX=on  SenseY=on  SenseZ=on  SenseXYZ=off  SenseRad=off  SenseAzim=off  SenseDist=off  SenseInc=off  SenseXDot=off  SenseYDot=off  SenseZDot=off  SenseXYZDot=off  SenseRadDot=off  SenseAzimDot=off  SenseDistDot=off  SenseIncDot=off  SenseXDDot=off  SenseYDDot=off  SenseZDDot=off  SenseXYZDDot=off  SenseRadDDot=off  SenseAzimDDot=off  SenseDistDDot=off  SenseIncDDot=off
  Foot : PMIOPort  Side=Left
  WorldFrame : PMIOPort  Port=2  Side=Right
  CartPos : Outport
  FootDeg : Outport  Port=2
  wires:
  PS-Simulink Converter/1 -> Bus Creator/3
  PS-Simulink Converter2/1 -> Bus Creator/2
  PS-Simulink Converter3/1 -> Bus Creator/1
  Bus Creator/1 -> CartPos/1
  PS-Simulink Converter1/1 -> QurtToDeg/1(q)
  QurtToDeg/3(Z_Yaw) -> Bus Creator1/3  "Z_Yaw"
  QurtToDeg/2(Y_Pitch) -> Bus Creator1/2  "Y_Pitch"
  QurtToDeg/1(X_Roll) -> Bus Creator1/1  "X_Roll"
  Bus Creator1/1 -> FootDeg/1
  connections:
  Foot/RConn1 -- Transform Sensor/LConn1
  WorldFrame/RConn1 -- Transform Sensor/RConn1
  PS-Simulink Converter/LConn1 -- Transform Sensor/RConn5
  PS-Simulink Converter3/LConn1 -- Transform Sensor/RConn3
  PS-Simulink Converter2/LConn1 -- Transform Sensor/RConn4
  PS-Simulink Converter1/LConn1 -- Transform Sensor/RConn2

== system PoleCart/Plant/Body/TibiaSensor ==
  Bus Creator : BusCreator  Inputs=3
  PS-Simulink Converter : nesl_utility/PS-Simulink Converter  PhysicalDomain=network_engine_domain  SubClassName=ps_output  LeftPortType=input  RightPortType=output  PseudoPeriodic=off  Frequencies=[]  VectorFormat=inherit  Unit=inherit  AffineConversion=off
  PS-Simulink Converter2 : nesl_utility/PS-Simulink Converter  PhysicalDomain=network_engine_domain  SubClassName=ps_output  LeftPortType=input  RightPortType=output  PseudoPeriodic=off  Frequencies=[]  VectorFormat=inherit  Unit=inherit  AffineConversion=off
  QurtToRad : Subsystem
  Scope1 : Scope
      settings: ActiveDisplayYMinimum=-115.26464605117451  ActiveDisplayYMaximum=70.275451311498813  DataLoggingVariableName=ScopeData3
  Transform Sensor : sm_lib/Frames and Transforms/Transform Sensor  MeasurementFrame=World  RotationSequence=ZYX  SenseAngle=off  SenseAxis=off  SenseQ=on  SenseR=off  SenseRotationSequence=off  SenseOmegaX=off  SenseOmegaY=off  SenseOmegaZ=off  SenseOmega=off  SenseQDot=off  SenseRDot=off  SenseRotationSequenceDot=off  SenseAlphaX=on  SenseAlphaY=off  SenseAlphaZ=off  SenseAlpha=off  SenseQDDot=off  SenseRDDot=off  SenseX=off  SenseY=off  SenseZ=off  SenseXYZ=off  SenseRad=off  SenseAzim=off  SenseDist=off  SenseInc=off  SenseXDot=off  SenseYDot=off  SenseZDot=off  SenseXYZDot=off  SenseRadDot=off  SenseAzimDot=off  SenseDistDot=off  SenseIncDot=off  SenseXDDot=off  SenseYDDot=off  SenseZDDot=off  SenseXYZDDot=off  SenseRadDDot=off  SenseAzimDDot=off  SenseDistDDot=off  SenseIncDDot=off
  WorldFrame : PMIOPort  Side=Left
  Tibia : PMIOPort  Port=2  Side=Right
  PoleRad : Outport
  PoleAcc : Outport  Port=2
  wires:
  PS-Simulink Converter/1 -> QurtToRad/1(q)
  QurtToRad/2(Y_Pitch) -> Bus Creator/2  "Y_Pitch"
  QurtToRad/3(Z_Yaw) -> Bus Creator/3  "Z_Yaw"
  QurtToRad/1(X_Roll) -> Bus Creator/1  "X_Roll"
  Bus Creator/1 -> PoleRad/1
  PS-Simulink Converter2/1 -> Scope1/1, PoleAcc/1
  connections:
  PS-Simulink Converter/LConn1 -- Transform Sensor/RConn2
  WorldFrame/RConn1 -- Transform Sensor/RConn1
  Tibia/RConn1 -- Transform Sensor/LConn1
  PS-Simulink Converter2/LConn1 -- Transform Sensor/RConn3

== system PoleCart/Plant/WorldFrame/Subsystem2 ==
  Mechanism Configuration : sm_lib/Utilities/Mechanism Configuration  UniformGravity=Constant  GravityVector=[0 0 -9.80665]  GravityVectorUnits=m/s^2  LinearizationDelta=0.001  JointModeTransitionNonlinearIterations=2
  Solver Configuration : nesl_utility/Solver Configuration  PhysicalDomain=network_engine_domain  SubClassName=solver  LeftPortType=input  RightPortType=generic  Tones=[]  Harmonics=[]  SimulateNoise=off  Profile=off  UseLocalSampling=off  EnableSwitchedLinearOptims=on  FrequencyDomain=off  UseCCode=off  RelTol=0.001  AbsTol=1e-06  MinStep=1e-09  ToWorkspace=off  RevertToSquareIcSolve=off  NumHomotopyIterations=100  PhasorMode=off  PhasorModeNumHarmonics=1  ConsistencySolver=NEWTON_XTOL_AFTER_FTOL  IndexReductionMethod=DerivativeReplacement  DoDC=off  ResidualTolerance=1e-09  ConsistencyTolSource=GLOBAL  ConsistencyAbsTol=0.001  ConsistencyRelTol=0.001  ConsistencyTolFactor=0.001  UseLocalSolver=off  LocalSolverChoice=NE_BACKWARD_EULER_ADVANCER  ResolveIndetEquations=on  FunctionEvalNumThread=1  LocalSolverSampleTime=0.001  DoFixedCost=off  MaxNonlinIter=3  MaxModeIter=2  ComputeImpulses=off  ImpulseIterations=2  LinearAlgebra=Sparse  LinearAlgebraNumThread=0  EquationFormulation=NE_TIME_EF  DelaysMemoryBudget=1024  AutomaticFiltering=on  FilteringTimeConstant=0.001  PartitionStorageMethod=AS_NEEDED  PartitionMemoryBudget=1024  PartitionMethod=FAST  MultibodyUseLocalSolver=off  MultibodyLocalSolverChoice=ODE1  MultibodyLocalSolverSampleTime=0.001
  World Frame : sm_lib/Frames and Transforms/World Frame
  WF : PMIOPort  Side=Right
  connections:
  World Frame/RConn1 -- WF/RConn1 -- Solver Configuration/RConn1 -- Mechanism Configuration/RConn1

== system PoleCart/Plant/Body/Subsystem/QurtToDeg ==
  q : Inport
  Demux : Demux
  Subsystem : Subsystem
  Subsystem1 : Subsystem
  Subsystem2 : Subsystem
  X_Roll : Outport
  Y_Pitch : Outport  Port=2
  Z_Yaw : Outport  Port=3
  wires:
  Demux/1 -> Subsystem2/1(w), Subsystem1/1(w), Subsystem/1(w)  "w"
  Demux/2 -> Subsystem2/2(x), Subsystem1/2(x), Subsystem/2(x)  "x"
  Demux/3 -> Subsystem2/3(y), Subsystem1/3(y), Subsystem/3(y)  "y"
  Demux/4 -> Subsystem2/4(z), Subsystem1/4(z), Subsystem/4(z)  "z"
  q/1 -> Demux/1
  Subsystem/1(Roll) -> X_Roll/1  "Roll"
  Subsystem1/1(Pitch) -> Y_Pitch/1  "Pitch"
  Subsystem2/1(Yaw) -> Z_Yaw/1  "Yaw"

== system PoleCart/Plant/Body/TibiaSensor/QurtToRad ==
  q : Inport
  Demux : Demux
  Subsystem : Subsystem
  Subsystem1 : Subsystem
  Subsystem2 : Subsystem
  X_Roll : Outport
  Y_Pitch : Outport  Port=2
  Z_Yaw : Outport  Port=3
  wires:
  Demux/1 -> Subsystem2/1(w), Subsystem1/1(w), Subsystem/1(w)  "w"
  Demux/2 -> Subsystem2/2(x), Subsystem1/2(x), Subsystem/2(x)  "x"
  Demux/3 -> Subsystem2/3(y), Subsystem1/3(y), Subsystem/3(y)  "y"
  Demux/4 -> Subsystem2/4(z), Subsystem1/4(z), Subsystem/4(z)  "z"
  q/1 -> Demux/1
  Subsystem/1(Roll) -> X_Roll/1  "Roll"
  Subsystem1/1(Pitch) -> Y_Pitch/1  "Pitch"
  Subsystem2/1(Yaw) -> Z_Yaw/1  "Yaw"

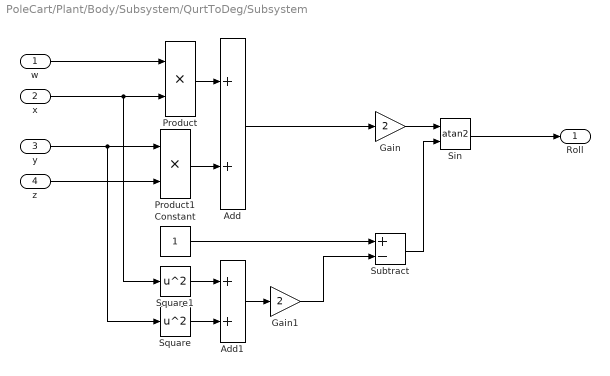
== system PoleCart/Plant/Body/Subsystem/QurtToDeg/Subsystem ==
  w : Inport
  x : Inport  Port=2
  y : Inport  Port=3
  z : Inport  Port=4
  Add : Sum
  Add1 : Sum
  Constant : Constant
  Gain : Gain  Gain=2
  Gain1 : Gain  Gain=2
  Product : Product
  Product1 : Product
  Sin : Trigonometry  Operator=atan2
  Square : Math  Operator=square
  Square1 : Math  Operator=square
  Subtract : Sum  Inputs=+-
  Roll : Outport
  wires:
  Subtract/1 -> Sin/2
  Constant/1 -> Subtract/1
  z/1 -> Product1/2
  y/1 -> Square/1, Product1/1
  Add/1 -> Gain/1
  Square/1 -> Add1/2
  Add1/1 -> Gain1/1
  Square1/1 -> Add1/1
  x/1 -> Square1/1, Product/2
  Gain/1 -> Sin/1
  Product/1 -> Add/1
  Product1/1 -> Add/2
  w/1 -> Product/1
  Sin/1 -> Roll/1
  Gain1/1 -> Subtract/2

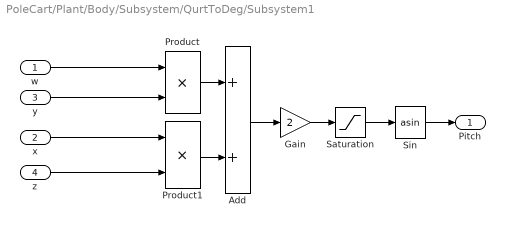
== system PoleCart/Plant/Body/Subsystem/QurtToDeg/Subsystem1 ==
  w : Inport
  x : Inport  Port=2
  y : Inport  Port=3
  z : Inport  Port=4
  Add : Sum
  Gain : Gain  Gain=2
  Product : Product
  Product1 : Product
  Saturation : Saturate  UpperLimit=1  LowerLimit=-1
  Sin : Trigonometry  Operator=asin
  Pitch : Outport
  wires:
  w/1 -> Product/1
  Product1/1 -> Add/2
  Product/1 -> Add/1
  Gain/1 -> Saturation/1
  Add/1 -> Gain/1
  z/1 -> Product1/2
  y/1 -> Product/2
  x/1 -> Product1/1
  Sin/1 -> Pitch/1
  Saturation/1 -> Sin/1

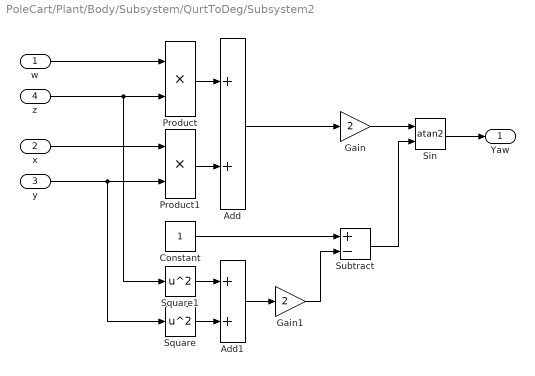
== system PoleCart/Plant/Body/Subsystem/QurtToDeg/Subsystem2 ==
  w : Inport
  x : Inport  Port=2
  y : Inport  Port=3
  z : Inport  Port=4
  Add : Sum
  Add1 : Sum
  Constant : Constant
  Gain : Gain  Gain=2
  Gain1 : Gain  Gain=2
  Product : Product
  Product1 : Product
  Sin : Trigonometry  Operator=atan2
  Square : Math  Operator=square
  Square1 : Math  Operator=square
  Subtract : Sum  Inputs=+-
  Yaw : Outport
  wires:
  Subtract/1 -> Sin/2
  Constant/1 -> Subtract/1
  Add/1 -> Gain/1
  Square/1 -> Add1/2
  Add1/1 -> Gain1/1
  Square1/1 -> Add1/1
  z/1 -> Square1/1, Product/2
  Gain/1 -> Sin/1
  Product/1 -> Add/1
  Product1/1 -> Add/2
  w/1 -> Product/1
  Sin/1 -> Yaw/1
  x/1 -> Product1/1
  y/1 -> Product1/2, Square/1
  Gain1/1 -> Subtract/2

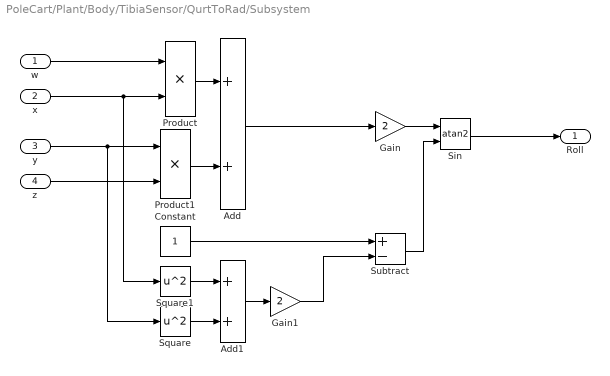
== system PoleCart/Plant/Body/TibiaSensor/QurtToRad/Subsystem ==
  w : Inport
  x : Inport  Port=2
  y : Inport  Port=3
  z : Inport  Port=4
  Add : Sum
  Add1 : Sum
  Constant : Constant
  Gain : Gain  Gain=2
  Gain1 : Gain  Gain=2
  Product : Product
  Product1 : Product
  Sin : Trigonometry  Operator=atan2
  Square : Math  Operator=square
  Square1 : Math  Operator=square
  Subtract : Sum  Inputs=+-
  Roll : Outport
  wires:
  Subtract/1 -> Sin/2
  Constant/1 -> Subtract/1
  z/1 -> Product1/2
  y/1 -> Square/1, Product1/1
  Add/1 -> Gain/1
  Square/1 -> Add1/2
  Add1/1 -> Gain1/1
  Square1/1 -> Add1/1
  x/1 -> Square1/1, Product/2
  Gain/1 -> Sin/1
  Product/1 -> Add/1
  Product1/1 -> Add/2
  w/1 -> Product/1
  Sin/1 -> Roll/1
  Gain1/1 -> Subtract/2

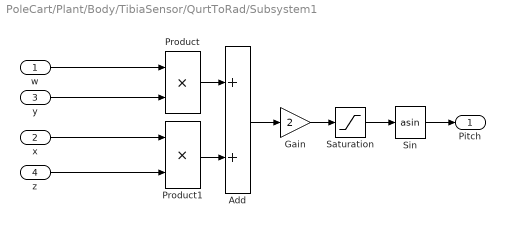
== system PoleCart/Plant/Body/TibiaSensor/QurtToRad/Subsystem1 ==
  w : Inport
  x : Inport  Port=2
  y : Inport  Port=3
  z : Inport  Port=4
  Add : Sum
  Gain : Gain  Gain=2
  Product : Product
  Product1 : Product
  Saturation : Saturate  UpperLimit=1  LowerLimit=-1
  Sin : Trigonometry  Operator=asin
  Pitch : Outport
  wires:
  w/1 -> Product/1
  Product1/1 -> Add/2
  Product/1 -> Add/1
  Gain/1 -> Saturation/1
  Add/1 -> Gain/1
  z/1 -> Product1/2
  y/1 -> Product/2
  x/1 -> Product1/1
  Sin/1 -> Pitch/1
  Saturation/1 -> Sin/1

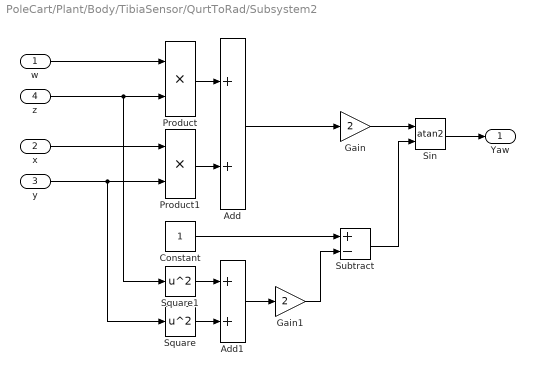
== system PoleCart/Plant/Body/TibiaSensor/QurtToRad/Subsystem2 ==
  w : Inport
  x : Inport  Port=2
  y : Inport  Port=3
  z : Inport  Port=4
  Add : Sum
  Add1 : Sum
  Constant : Constant
  Gain : Gain  Gain=2
  Gain1 : Gain  Gain=2
  Product : Product
  Product1 : Product
  Sin : Trigonometry  Operator=atan2
  Square : Math  Operator=square
  Square1 : Math  Operator=square
  Subtract : Sum  Inputs=+-
  Yaw : Outport
  wires:
  Subtract/1 -> Sin/2
  Constant/1 -> Subtract/1
  Add/1 -> Gain/1
  Square/1 -> Add1/2
  Add1/1 -> Gain1/1
  Square1/1 -> Add1/1
  z/1 -> Square1/1, Product/2
  Gain/1 -> Sin/1
  Product/1 -> Add/1
  Product1/1 -> Add/2
  w/1 -> Product/1
  Sin/1 -> Yaw/1
  x/1 -> Product1/1
  y/1 -> Product1/2, Square/1
  Gain1/1 -> Subtract/2
